simulink model "control_system_lin_lin"  (R2025b)
settings: Solver=FixedStepAuto  StartTime=0.0  StopTime=10.0  FixedStep=0.01  RelTol=1e-3
values from neighbouring files (symbols this model uses):
  A = double(J_xeq_ueq)    [init_control_system_lin_lin.m]
  B = [0 1]'    [init_control_system_lin_lin.m]
  K = -place(A,B,[-1 -1.1])    [init_control_system_lin_lin.m]
  ueq = 0    [init_control_system_lin_lin.m]
  x0 = [1 1.5]'    [init_control_system_lin_lin.m]
  xeq = S2    [init_control_system_lin_lin.m]
settings Model: Creator=ricca  LastModifiedBy=ricca

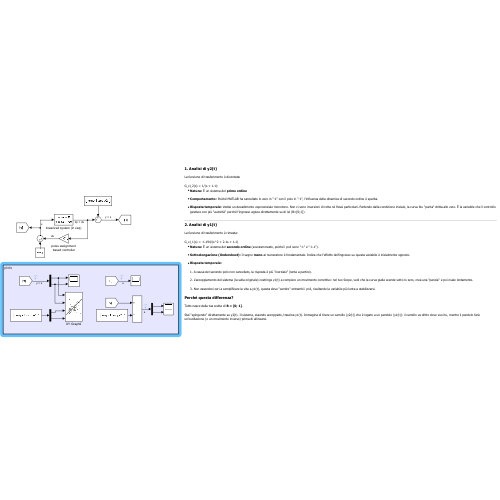
[thumbnail: Simulink's stored preview of the top-level diagram]
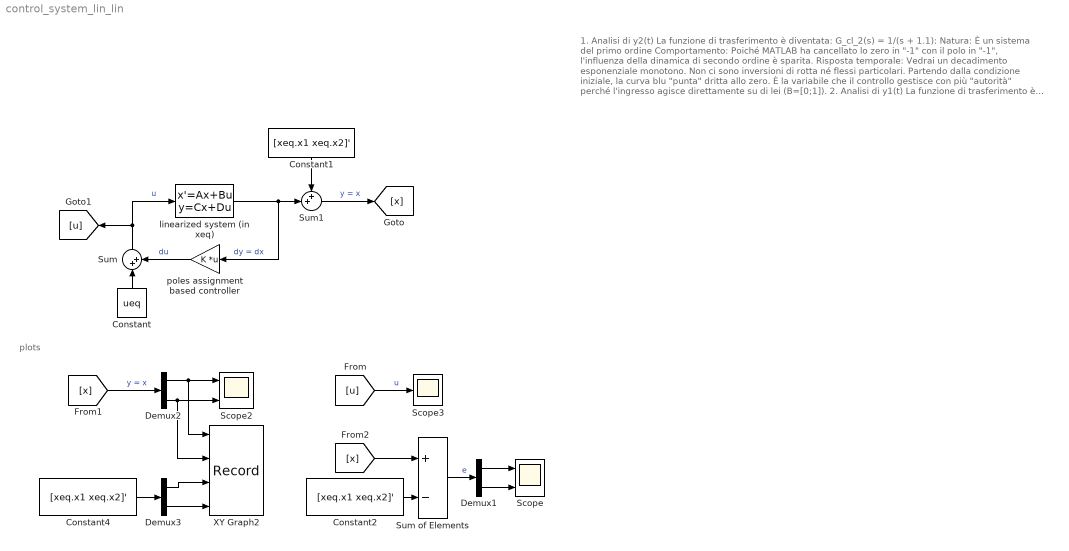
== system control_system_lin_lin ==
  note: 1. Analisi di y2(t)
      | La funzione di trasferimento è diventata:
      | G_cl_2(s) = 1/(s + 1.1):
      | Natura: È un sistema del primo ordine
      | Comportamento: Poiché MATLAB ha cancellato lo zero in "-1" con il polo in "-1", l'influenza della dinamica di secondo ordine è sparita.
      | Risposta temporale: Vedrai un decadimento esponenziale monotono. Non ci sono inversioni di rotta né flessi particolari. Partendo dalla condizione iniziale, la curva blu "punta" dritta allo zero. È la variabile che il controllo gestisce con più "autorità" perché l'ingresso agisce direttamente su di lei (B=[0;1]).
      | 2. Analisi di y1(t)
      | La funzione di trasferimento è rimasta:
      | G_cl_1(s) = -1.194/(s^2 + 2.1s + 1.1)
      | Natura: È un sistema del secondo ordine (sovrasmorzato, poiché i poli sono "-1" e "-1.1").
      | Sottoelongazione (Undershoot): Il segno meno al numeratore è fondamentale. Indica che l'effetto dell'ingresso su questa variabile è inizialmente opposto.
      | Risposta temporale:
      | 1. A causa del secondo polo non cancellato, la risposta è più "inerziale" (lenta a partire).
      | 2. L'accoppiamento del sistema (la sella originale) costringe y1(t) a compiere un movimento correttivo: nel tuo Scope, vedi che la curva gialla scende sotto lo zero, crea una "pancia" e poi risale lentamente.
      | 3. Non essendoci zeri a semplificare la vita a y1(t), questa deve "sentire" entrambi i poli, risultando la variabile più lenta a stabilizzarsi.
      | Perché questa differenza?
      | Tutto nasce dalla tua scelta di B = [0; 1] .
      | Stai "spingendo" direttamente su y2(t). Il sistema, essendo accoppiato, trascina y1(t). Immagina di tirare un carrello (y2(t)) che è legato a un pendolo (y1(t)): il carrello va dritto dove vuoi tu, mentre il pendolo farà un'oscillazione (o un movimento inverso) prima di allinearsi.
  note: plots
  Constant : Constant  Value=ueq
  Constant1 : Constant  Value=[xeq.x1 xeq.x2]'
  Constant2 : Constant  Value=[xeq.x1 xeq.x2]'
  Constant4 : Constant  Value=[xeq.x1 xeq.x2]'
  Demux1 : Demux  Outputs=2
  Demux2 : Demux  Outputs=2
  Demux3 : Demux  Outputs=2
  Scope : Scope  NumInputPorts=2
      settings: ActiveDisplayYMinimum=-2.1110906236978666  ActiveDisplayYMaximum=2.1840346802383825
  Scope2 : Scope  NumInputPorts=2
      settings: ActiveDisplayYMinimum=0.59700937630213358  ActiveDisplayYMaximum=4.8921346802383825  DataLoggingVariableName=ScopeData2
  Scope3 : Scope
      settings: ActiveDisplayYMinimum=-3.0982249093162668  ActiveDisplayYMaximum=1.2143219033221408  DataLoggingVariableName=ScopeData3
  Sum : Sum  Inputs=|++
  Sum of Elements : Sum  Inputs=+-
  Sum1 : Sum  Inputs=++|
  XY Graph2 : Record  NumPorts=4.0  FileSettingsInternal="{\"entries\":[{\"content\":{\"excelSettings\":{\"content\":{},\"type\":\"Streamout.ExcelSettings\"},\"parquetSettings\":{\"content\":{},\"type\":\"Streamout.ParquetSettings\"}},\"type\":\"Streamout.FileSettingStorage\",\"uuid\":\"\"}],\"packageUris\":[\"http:\\/\\/schema.mathworks.com\\/mf0\\/streamout_blocks\\/R2020a\"],\"version\":\"1.0\"}"  FrameSettings=[0, 0, 0, 0]  Layout=[1 1]  SignalsInternal="{\"entries\":[{\"content\":{\"signals\":[{\"content\":{\"blockPath\":[],\"dimensions\":[1],\"domain\":\"\",\"lineColor\":\"#139fff\",\"plots\":[ 1 ],\"port\":1,\"sid\":[\"\"],\"signalID\":1,\"signalName\":\"Demux2:1\"},\"type\":\"RecordBlkView.Signal\",\"uuid\":\"\"},{\"content\":{\"blockPath\":[],\"dimensions\":[1],\"domain\":\"\",\"lineColor\":\"#139fff\",\"plots\":[ 1 ],\"port\":2,\"sid\":[\"\"],\"signalID\":2,\"signalName\":\"Demux2:2\"},\"type\":\"RecordBlkView.Signal\",\"uuid\":\"\"},{\"content\":{\"blockPath\":[],\"dimensions\":[1],\"domain\":\"\",\"lineColor\":\"#a2142f\",\"lineWidth\":20,\"plots\":[ 1 ],\"port\":3,\"sid\":[\"\"],\"signalID\":3,\"signalName\":\"Demux3:1\"},\"type\":\"RecordBlkView.Signal\",\"uuid\":\"\"},{\"content\":{\"blockPath\":[],\"dimensions\":[1],\"domain\":\"\",\"lineColor\":\"#a2142f\",\"lineWidth\":20,\"plots\":[ 1 ],\"port\":4,\"sid\":[\"\"],\"signalID\":4,\"signalName\":\"Demux3:2\"},\"type\":\"RecordBlkView.Signal\",\"uuid\":\"\"}]},\"type\":\"RecordBlkView.InputSignals\",\"uuid\":\"\"}],\"packageUris\":[\"http:\\/\\/schema.mathworks.com\\/mf0\\/streamout_blocks\\/R2020a\"],\"version\":\"1.0\"}"  VisualizationBindings="{\"xyplotplugin\":{\"info\":[{\"series\":[{\"bindingParametersList\":[{\"parameter\":\"X-Axis\",\"signalID\":3,\"signalName\":\"Demux3:1\"},{\"parameter\":\"Y-Axis\",\"signalID\":4,\"signalName\":\"Demux3:2\"}],\"seriesID\":0},{\"bindingParametersList\":[{\"parameter\":\"X-Axis\",\"signalID\":1,\"signalName\":\"Demux2:1\"},{\"parameter\":\"Y-Axis\",\"signalID\":2,\"signalName\":\"Demux2:2\"}],\"seriesID\":1}],\"subplotID\":1}]}}"  CompatibilityTag=XY
  linearized system (in xeq) : StateSpace  A=A  B=B  C=eye(2)  D=[0 0]'  InitialCondition=[ 0 - (xeq.x1 - x0(1)), 0 - (xeq.x2 - x0(2))]'
  poles assignment based controller : Gain  Gain=K  Multiplication=Matrix(K*u)
  wires:
  Sum1/1 -> [x]  "y = x"
  poles assignment based controller/1 -> Sum/2  "du"
  Constant/1 -> Sum/1
  Sum/1 -> [u], linearized system (in xeq)/1  "u"
  linearized system (in xeq)/1 -> poles assignment based controller/1, Sum1/2  "dy = dx"
  Constant1/1 -> Sum1/1
  Sum of Elements/1 -> Demux1/1  "e"
  Demux1/2 -> Scope/2
  Demux1/1 -> Scope/1
  [u] -> Scope3/1  "u"
  [x] -> Demux2/1  "y = x"
  Demux3/2 -> XY Graph2/4
  Demux2/1 -> XY Graph2/1, Scope2/1
  Constant2/1 -> Sum of Elements/2
  Demux2/2 -> XY Graph2/2, Scope2/2
  Constant4/1 -> Demux3/1
  Demux3/1 -> XY Graph2/3
  [x] -> Sum of Elements/1
